simulink model "KinematicsComplianceIndependentSuspensionFront"  (R2026b)
settings: Solver=VariableStepAuto
undefined symbols (not defined in the file): PlntVehCGHgtAxl, PlntVehTrckWdth, PlntWhlNumFrnt
libraries: autolibsharedcommon x6, autolibutils x3, matrix_library x2, vehdynlibsuspension x1
(part 1 of 2)
settings Model: ModifiedByFormat=The MathWorks, Inc.  Creator=The MathWorks, Inc.  LastModifiedBy=The MathWorks, Inc.
settings OptimizationCC: ReuseModelBlockBuffer=off
settings DebuggingCC: SubsystemReferenceDiagnosticForUnitTest=warning
settings RTWCC: LargeConstantGeneration=WriteOnlyDNNConstantsToDataFiles

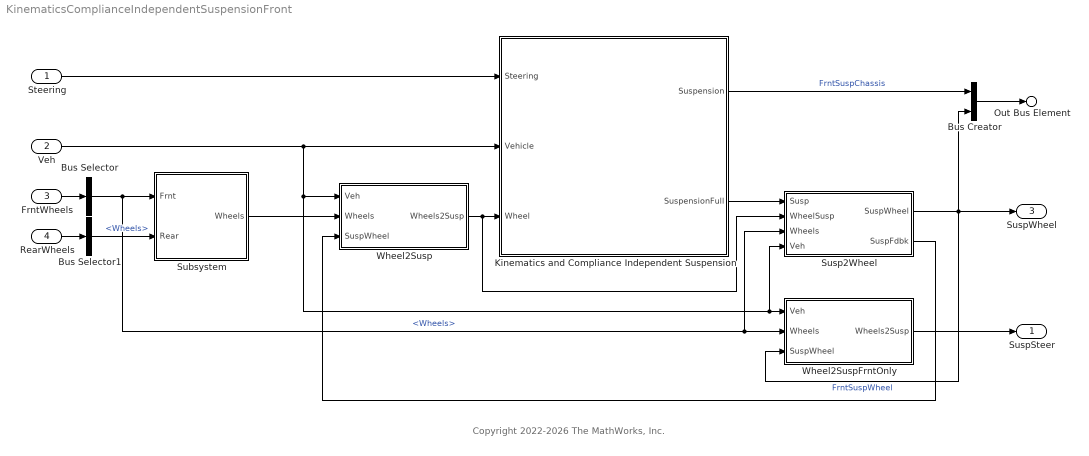
== system KinematicsComplianceIndependentSuspensionFront ==
  note: Copyright 2022-2026 The MathWorks, Inc.
  Steering : Inport
  Veh : Inport  Port=2
  FrntWheels : Inport  Port=3
  RearWheels : Inport  Port=4
  Bus Creator : BusCreator  Inputs=2
  Bus Selector : BusSelector  OutputSignals=Wheels
  Bus Selector1 : BusSelector  OutputSignals=Wheels
  Kinematics and Compliance Independent Suspension : Subsystem  VariantControl=Kinematics and Compliance Independent Suspension
      mask Display: image('suspkandc.png');
  Subsystem : Subsystem
  Susp2Wheel : Subsystem
  Wheel2Susp : Subsystem
  Wheel2SuspFrntOnly : Subsystem
  SuspSteer : Outport
  Out Bus Element : Outport  Port=2  PortName=FrntSusp
  SuspWheel : Outport  Port=3
  wires:
  Veh/1 -> Kinematics and Compliance Independent Suspension/2(Vehicle), Susp2Wheel/4(Veh), Wheel2SuspFrntOnly/1(Veh), Wheel2Susp/1(Veh)
  Susp2Wheel/1(SuspWheel) -> Wheel2SuspFrntOnly/3(SuspWheel), Bus Creator/2, SuspWheel/1  "FrntSuspWheel"
  Subsystem/1(Wheels) -> Wheel2Susp/2(Wheels)
  Kinematics and Compliance Independent Suspension/1(Suspension) -> Bus Creator/1  "FrntSuspChassis"
  Wheel2Susp/1(Wheels2Susp) -> Susp2Wheel/2(WheelSusp), Kinematics and Compliance Independent Suspension/3(Wheel)
  Steering/1 -> Kinematics and Compliance Independent Suspension/1(Steering)
  Bus Selector/1 -> Susp2Wheel/3(Wheels), Wheel2SuspFrntOnly/2(Wheels), Subsystem/1(Frnt)  "<Wheels>"
  RearWheels/1 -> Bus Selector1/1
  FrntWheels/1 -> Bus Selector/1
  Bus Selector1/1 -> Subsystem/2(Rear)  "<Wheels>"
  Bus Creator/1 -> Out Bus Element/1
  Susp2Wheel/2(SuspFdbk) -> Wheel2Susp/3(SuspWheel)
  Kinematics and Compliance Independent Suspension/2(SuspensionFull) -> Susp2Wheel/1(Susp)
  Wheel2SuspFrntOnly/1(Wheels2Susp) -> SuspSteer/1

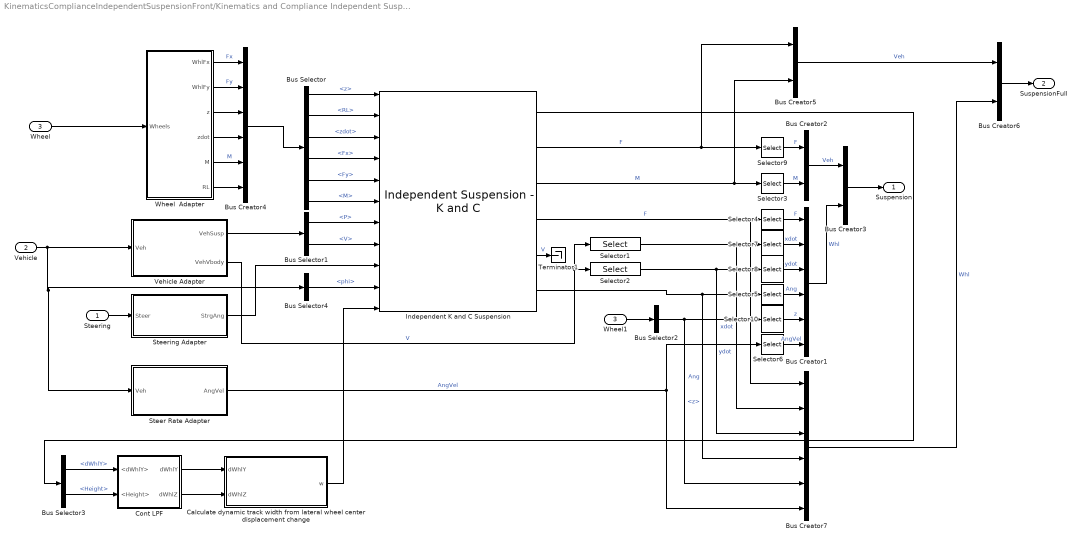
== system KinematicsComplianceIndependentSuspensionFront/Kinematics and Compliance Independent Suspension ==
  Steering : Inport
  Vehicle : Inport  Port=2
  Wheel : Inport  Port=3
  Bus Creator1 : BusCreator  Inputs=6
  Bus Creator{2..3,5..6} (4 alike) : BusCreator  Inputs=2
  Bus Creator4 : BusCreator  Inputs=6
  Bus Creator7 : BusCreator  Inputs=6
  Bus Selector : BusSelector  OutputSignals=z,RL,zdot,Fx,Fy,M
  Bus Selector1 : BusSelector  OutputSignals=P,V
  Bus Selector2 : BusSelector  OutputSignals=SuspFrame.z
  Bus Selector3 : BusSelector  OutputSignals=dWhlY,Height
  Bus Selector4 : BusSelector  OutputSignals=InertFrm.Cg.Ang.phi
  Calculate dynamic track width from lateral wheel center displacement change : Subsystem  mask{w=PlntVehTrckWdth}
      mask prompts: w "vdynblks:vehdynVehBody6Dof:blkPrm_w"
      mask DialogControl w Prompt: Track widths [front, rear], w [m]:
  Cont LPF : Subsystem
  Independent K and C Suspension : vehdynlibsuspension/Independent Suspension - K and C  ActiveDampEn=off  NumAxl=2  NumWhlsByAxl=[2 2]  StrgEnByAxl=[1 0]  AntiSwayEnByAxl=[1 1]  WhlNumVec="[1  2  1  2]"  AxleNumVec="[1  1  2  2]"  SuspTypesByAxle="[1  1]"  SuspImage=suspkandc.png  IdealSuspEn=on  IdealSuspAxles="[1  2]"  tanTheta_FL=[0 0 0]  tanTheta_FR=[0 0 0]  tanTheta_RL=[0 0 0]  tanTheta_RR=[0 0 0]  SteerSign=1  LongitudinalSign=1  LateralSign=1  VerticalSign=1  WhlMzSign=1  tanTheta_SVSA_WC_FL=1  tanTheta_SVSA_WC_FR=1  tanTheta_SVSA_WC_RL=1  tanTheta_SVSA_WC_RR=1  tanTheta_SVSA_CP_FL=1  tanTheta_SVSA_CP_FR=1  tanTheta_SVSA_CP_RL=1  tanTheta_SVSA_CP_RR=1  SuspType=Independent front and rear  DrivetrainType=FWD  StrPlusDirection=Right  XPlusDirection=Front  YPlusDirection=Right  ZPlusDirection=Up  WhlMzDirection=Counter-clockwise  ShockType=Constant  ShckFrcVsCompRate=PlntSpKCShckFrcVsCompRate  MotRatios=PlntSpKCMotRatios  BumpSteer=PlntSpKCBumpSteer  BumpCamber=PlntSpKCBumpCamber  BumpCaster=PlntSpKCBumpCaster  LatWhlCtrDisp=PlntSpKCLatWhlCtrDisp  LngWhlCtrDisp=PlntSpKCLngWhlCtrDisp  NrmlWhlRates=PlntSpKCNrmlWhlRates  NrmlWhlFrcOff=PlntSpKCNrmlWhlFrcOff  RollSteer=[0 0 0 0]  RollCamber=[0 0 0 0]  RollCaster=[0 0 0 0]  RollStiffArb=PlntSpKCRollStiffArb  RollStiffNoArb=PlntSpKCRollStiffNoArb  RollStiffArbFrnt=800  RollStiffNoArbFrnt=0  RollStiffNoTwstRear=0  CambVsSteerAng=PlntSpKCCambVsSteerAng  CastVsSteerAng=PlntSpKCCastVsSteerAng  LngSteerCompl=PlntSpKCLngSteerCompl  LngCambCompl=PlntSpKCLngCambCompl  LngCastCompl=PlntSpKCLngCastCompl  LngWhlCtrCompl=PlntSpKCLngWhlCtrCompl  LatWhlCtrComplLng=PlntSpKCLatWhlCtrComplLng  LatSteerCompl=PlntSpKCLatSteerCompl  LatCambCompl=PlntSpKCLatCambCompl  LatWhlCtrComplLat=PlntSpKCLatWhlCtrComplLat  LatSteerComplOpp=PlntSpKCLatSteerCompl  LatCambComplOpp=PlntSpKCLatCambCompl  LatWhlCtrComplLatOpp=PlntSpKCLatWhlCtrComplLat  AlgnTrqSteerCompl=PlntSpKCAlgnTrqSteerCompl  AlgnTrqCambCompl=PlntSpKCAlgnTrqCambCompl  VrtLdTrnsfr=PlntSpKCVrtLdTrnsfr  LatSteerComplPar=struct('FL',[-2. -1.;0 0;2. 1.],'FR',[-2. 1.;0 0;2. -1.],'RL',[-2. -1.;0 0;2. 1.],'RR',[-2. 1.;0 0;2. -1.])  LatCambComplPar=struct('FL',[-2. -1.;0 0;2. 1.],'FR',[-2. 1.;0 0;2. -1.],'RL',[-2. -1.;0 0;2. 1.],'RR',[-2. 1.;0 0;2. -1.])  LatWhlCtrComplLatPar=struct('FL',[-2. -5.;0 0;2. 5.],'FR',[-2. 5.;0 0;2. -5.],'RL',[-2. -5.;0 0;2. 5.],'RR',[-2. 5.;0 0;2. -5.])  StatToe=PlntSpKCStatToe  StatCamber=PlntSpKCStatCamber  StatCaster=PlntSpKCStatCaster  StatLdWhlR=PlntSpStatLdWhlR  MappedSuspEn=off  RollParamEn=off
  Selector1 : Selector  NumberOfDimensions=2  IndexOptions=Index vector (dialog),Select all  Indices=1,1  OutputSizes=1,1
  Selector10 : Selector  InputPortWidth=4  IndexOptions=Index vector (dialog)  Indices=[1 2]  OutputSizes=1
  Selector2 : Selector  NumberOfDimensions=2  IndexOptions=Index vector (dialog),Select all  Indices=2,1  OutputSizes=1,1
  Selector{3..6,9} (5 alike) : Selector  NumberOfDimensions=2  InputPortWidth=4  IndexOptions=Index vector (dialog),Index vector (dialog)  Indices=[1 2 3],[1 2]  OutputSizes=1,1
  Selector7 : Selector  InputPortWidth=4  IndexOptions=Index vector (dialog)  Indices=[1 2]  OutputSizes=1
  Selector8 : Selector  InputPortWidth=4  IndexOptions=Index vector (dialog)  Indices=[1 2]  OutputSizes=1
  Steer Rate Adapter : Subsystem
  Steering Adapter : Subsystem
  Terminator1 : Terminator
  Vehicle Adapter : Subsystem
  Wheel  Adapter : Subsystem
  Wheel1 : InportShadow  Port=3
  Suspension : Outport  VectorParamsAs1DForOutWhenUnconnected=off
  SuspensionFull : Outport  Port=2  VectorParamsAs1DForOutWhenUnconnected=off
  wires:
  Bus Creator6/1 -> SuspensionFull/1
  Bus Creator7/1 -> Bus Creator6/2  "Whl"
  Bus Creator5/1 -> Bus Creator6/1  "Veh"
  Selector6/1 -> Bus Creator1/6  "AngVel"
  Selector10/1 -> Bus Creator1/5  "z"
  Selector5/1 -> Bus Creator1/4  "Ang"
  Selector8/1 -> Bus Creator1/3  "ydot"
  Selector7/1 -> Bus Creator1/2  "xdot"
  Selector4/1 -> Bus Creator1/1  "F"
  Selector3/1 -> Bus Creator2/2  "M"
  Selector9/1 -> Bus Creator2/1  "F"
  Bus Creator3/1 -> Suspension/1
  Bus Creator1/1 -> Bus Creator3/2  "Whl"
  Bus Selector1/2 -> Independent K and C Suspension/8  "<V>"
  Bus Selector/6 -> Independent K and C Suspension/6  "<M>"
  Bus Selector/5 -> Independent K and C Suspension/5  "<Fy>"
  Steering/1 -> Steering Adapter/1(Steer)
  Bus Selector/3 -> Independent K and C Suspension/3  "<zdot>"
  Bus Selector/4 -> Independent K and C Suspension/4  "<Fx>"
  Vehicle/1 -> Vehicle Adapter/1(Veh), Bus Selector4/1, Steer Rate Adapter/1(Veh)
  Vehicle Adapter/1(VehSusp) -> Bus Selector1/1
  Independent K and C Suspension/3 -> Selector3/1, Bus Creator5/2  "M"
  Wheel  Adapter/2(WhlFy) -> Bus Creator4/2  "Fy"
  Wheel  Adapter/1(WhlFx) -> Bus Creator4/1  "Fx"
  Wheel/1 -> Wheel  Adapter/1(Wheels)
  Wheel  Adapter/3(z) -> Bus Creator4/3
  Wheel  Adapter/4(zdot) -> Bus Creator4/4
  Wheel  Adapter/5(M) -> Bus Creator4/5  "M"
  Wheel  Adapter/6(RL) -> Bus Creator4/6
  Bus Selector/2 -> Independent K and C Suspension/2  "<RL>"
  Selector1/1 -> Selector7/1, Bus Creator7/2  "xdot"
  Selector2/1 -> Selector8/1, Bus Creator7/3  "ydot"
  Bus Selector1/1 -> Independent K and C Suspension/7  "<P>"
  Bus Selector/1 -> Independent K and C Suspension/1  "<z>"
  Independent K and C Suspension/4 -> Selector4/1, Bus Creator7/1  "F"
  Independent K and C Suspension/6 -> Selector5/1, Bus Creator7/4  "Ang"
  Vehicle Adapter/2(VehVbody) -> Selector1/1, Selector2/1  "V"
  Independent K and C Suspension/2 -> Selector9/1, Bus Creator5/1  "F"
  Bus Creator2/1 -> Bus Creator3/1  "Veh"
  Bus Creator4/1 -> Bus Selector/1
  Steer Rate Adapter/1(AngVel) -> Selector6/1, Bus Creator7/6  "AngVel"
  Steering Adapter/1(StrgAng) -> Independent K and C Suspension/9
  Independent K and C Suspension/1 -> Bus Selector3/1
  Independent K and C Suspension/5 -> Terminator1/1  "V"
  Bus Selector2/1 -> Selector10/1, Bus Creator7/5  "<z>"
  Wheel1/1 -> Bus Selector2/1
  Bus Selector4/1 -> Independent K and C Suspension/10  "<phi>"
  Calculate dynamic track width from lateral wheel center displacement change/1(w) -> Independent K and C Suspension/11
  Bus Selector3/1 -> Cont LPF/1(<dWhlY>)  "<dWhlY>"
  Bus Selector3/2 -> Cont LPF/2(<Height>)  "<Height>"
  Cont LPF/1(dWhlY) -> Calculate dynamic track width from lateral wheel center displacement change/1(dWhlY)
  Cont LPF/2(dWhlZ) -> Calculate dynamic track width from lateral wheel center displacement change/2(dWhlZ)

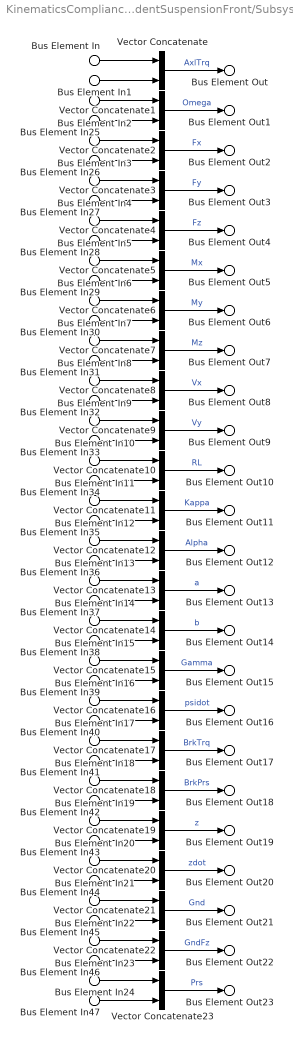
== system KinematicsComplianceIndependentSuspensionFront/Subsystem ==
  Bus Element In : Inport  PortName=Frnt  Element=AxlTrq
  Bus Element In2 : Inport  PortName=Frnt  Element=Omega
  Bus Element In3 : Inport  PortName=Frnt  Element=Fx
  Bus Element In4 : Inport  PortName=Frnt  Element=Fy
  Bus Element In5 : Inport  PortName=Frnt  Element=Fz
  Bus Element In6 : Inport  PortName=Frnt  Element=Mx
  Bus Element In7 : Inport  PortName=Frnt  Element=My
  Bus Element In8 : Inport  PortName=Frnt  Element=Mz
  Bus Element In9 : Inport  PortName=Frnt  Element=Vx
  Bus Element In10 : Inport  PortName=Frnt  Element=Vy
  Bus Element In11 : Inport  PortName=Frnt  Element=RL
  Bus Element In12 : Inport  PortName=Frnt  Element=Kappa
  Bus Element In13 : Inport  PortName=Frnt  Element=Alpha
  Bus Element In14 : Inport  PortName=Frnt  Element=a
  Bus Element In15 : Inport  PortName=Frnt  Element=b
  Bus Element In16 : Inport  PortName=Frnt  Element=Gamma
  Bus Element In17 : Inport  PortName=Frnt  Element=psidot
  Bus Element In18 : Inport  PortName=Frnt  Element=BrkTrq
  Bus Element In19 : Inport  PortName=Frnt  Element=BrkPrs
  Bus Element In20 : Inport  PortName=Frnt  Element=z
  Bus Element In21 : Inport  PortName=Frnt  Element=zdot
  Bus Element In22 : Inport  PortName=Frnt  Element=Gnd
  Bus Element In23 : Inport  PortName=Frnt  Element=GndFz
  Bus Element In24 : Inport  PortName=Frnt  Element=Prs
  Bus Element In1 : Inport  Port=2  PortName=Rear  Element=AxlTrq
  Bus Element In25 : Inport  Port=2  PortName=Rear  Element=Omega
  Bus Element In26 : Inport  Port=2  PortName=Rear  Element=Fx
  Bus Element In27 : Inport  Port=2  PortName=Rear  Element=Fy
  Bus Element In28 : Inport  Port=2  PortName=Rear  Element=Fz
  Bus Element In29 : Inport  Port=2  PortName=Rear  Element=Mx
  Bus Element In30 : Inport  Port=2  PortName=Rear  Element=My
  Bus Element In31 : Inport  Port=2  PortName=Rear  Element=Mz
  Bus Element In32 : Inport  Port=2  PortName=Rear  Element=Vx
  Bus Element In33 : Inport  Port=2  PortName=Rear  Element=Vy
  Bus Element In34 : Inport  Port=2  PortName=Rear  Element=RL
  Bus Element In35 : Inport  Port=2  PortName=Rear  Element=Kappa
  Bus Element In36 : Inport  Port=2  PortName=Rear  Element=Alpha
  Bus Element In37 : Inport  Port=2  PortName=Rear  Element=a
  Bus Element In38 : Inport  Port=2  PortName=Rear  Element=b
  Bus Element In39 : Inport  Port=2  PortName=Rear  Element=Gamma
  Bus Element In40 : Inport  Port=2  PortName=Rear  Element=psidot
  Bus Element In41 : Inport  Port=2  PortName=Rear  Element=BrkTrq
  Bus Element In42 : Inport  Port=2  PortName=Rear  Element=BrkPrs
  Bus Element In43 : Inport  Port=2  PortName=Rear  Element=z
  Bus Element In44 : Inport  Port=2  PortName=Rear  Element=zdot
  Bus Element In45 : Inport  Port=2  PortName=Rear  Element=Gnd
  Bus Element In46 : Inport  Port=2  PortName=Rear  Element=GndFz
  Bus Element In47 : Inport  Port=2  PortName=Rear  Element=Prs
  Vector Concatenate{,1..23} (24 alike) : Concatenate
  Bus Element Out : Outport  PortName=Wheels  Element=AxlTrq
  Bus Element Out1 : Outport  PortName=Wheels  Element=Omega
  Bus Element Out2 : Outport  PortName=Wheels  Element=Fx
  Bus Element Out3 : Outport  PortName=Wheels  Element=Fy
  Bus Element Out4 : Outport  PortName=Wheels  Element=Fz
  Bus Element Out5 : Outport  PortName=Wheels  Element=Mx
  Bus Element Out6 : Outport  PortName=Wheels  Element=My
  Bus Element Out7 : Outport  PortName=Wheels  Element=Mz
  Bus Element Out8 : Outport  PortName=Wheels  Element=Vx
  Bus Element Out9 : Outport  PortName=Wheels  Element=Vy
  Bus Element Out10 : Outport  PortName=Wheels  Element=RL
  Bus Element Out11 : Outport  PortName=Wheels  Element=Kappa
  Bus Element Out12 : Outport  PortName=Wheels  Element=Alpha
  Bus Element Out13 : Outport  PortName=Wheels  Element=a
  Bus Element Out14 : Outport  PortName=Wheels  Element=b
  Bus Element Out15 : Outport  PortName=Wheels  Element=Gamma
  Bus Element Out16 : Outport  PortName=Wheels  Element=psidot
  Bus Element Out17 : Outport  PortName=Wheels  Element=BrkTrq
  Bus Element Out18 : Outport  PortName=Wheels  Element=BrkPrs
  Bus Element Out19 : Outport  PortName=Wheels  Element=z
  Bus Element Out20 : Outport  PortName=Wheels  Element=zdot
  Bus Element Out21 : Outport  PortName=Wheels  Element=Gnd
  Bus Element Out22 : Outport  PortName=Wheels  Element=GndFz
  Bus Element Out23 : Outport  PortName=Wheels  Element=Prs
  wires:
  Vector Concatenate23/1 -> Bus Element Out23/1  "Prs"
  Vector Concatenate22/1 -> Bus Element Out22/1  "GndFz"
  Vector Concatenate21/1 -> Bus Element Out21/1  "Gnd"
  Vector Concatenate20/1 -> Bus Element Out20/1  "zdot"
  Vector Concatenate19/1 -> Bus Element Out19/1  "z"
  Vector Concatenate18/1 -> Bus Element Out18/1  "BrkPrs"
  Vector Concatenate17/1 -> Bus Element Out17/1  "BrkTrq"
  Vector Concatenate16/1 -> Bus Element Out16/1  "psidot"
  Vector Concatenate15/1 -> Bus Element Out15/1  "Gamma"
  Vector Concatenate14/1 -> Bus Element Out14/1  "b"
  Vector Concatenate13/1 -> Bus Element Out13/1  "a"
  Vector Concatenate12/1 -> Bus Element Out12/1  "Alpha"
  Vector Concatenate11/1 -> Bus Element Out11/1  "Kappa"
  Vector Concatenate10/1 -> Bus Element Out10/1  "RL"
  Vector Concatenate9/1 -> Bus Element Out9/1  "Vy"
  Vector Concatenate8/1 -> Bus Element Out8/1  "Vx"
  Vector Concatenate7/1 -> Bus Element Out7/1  "Mz"
  Vector Concatenate6/1 -> Bus Element Out6/1  "My"
  Vector Concatenate5/1 -> Bus Element Out5/1  "Mx"
  Vector Concatenate4/1 -> Bus Element Out4/1  "Fz"
  Vector Concatenate3/1 -> Bus Element Out3/1  "Fy"
  Vector Concatenate2/1 -> Bus Element Out2/1  "Fx"
  Vector Concatenate1/1 -> Bus Element Out1/1  "Omega"
  Vector Concatenate/1 -> Bus Element Out/1  "AxlTrq"
  Bus Element In47/1 -> Vector Concatenate23/2
  Bus Element In24/1 -> Vector Concatenate23/1
  Bus Element In46/1 -> Vector Concatenate22/2
  Bus Element In23/1 -> Vector Concatenate22/1
  Bus Element In45/1 -> Vector Concatenate21/2
  Bus Element In22/1 -> Vector Concatenate21/1
  Bus Element In44/1 -> Vector Concatenate20/2
  Bus Element In21/1 -> Vector Concatenate20/1
  Bus Element In43/1 -> Vector Concatenate19/2
  Bus Element In20/1 -> Vector Concatenate19/1
  Bus Element In42/1 -> Vector Concatenate18/2
  Bus Element In19/1 -> Vector Concatenate18/1
  Bus Element In41/1 -> Vector Concatenate17/2
  Bus Element In18/1 -> Vector Concatenate17/1
  Bus Element In40/1 -> Vector Concatenate16/2
  Bus Element In17/1 -> Vector Concatenate16/1
  Bus Element In39/1 -> Vector Concatenate15/2
  Bus Element In16/1 -> Vector Concatenate15/1
  Bus Element In38/1 -> Vector Concatenate14/2
  Bus Element In15/1 -> Vector Concatenate14/1
  Bus Element In37/1 -> Vector Concatenate13/2
  Bus Element In14/1 -> Vector Concatenate13/1
  Bus Element In36/1 -> Vector Concatenate12/2
  Bus Element In13/1 -> Vector Concatenate12/1
  Bus Element In35/1 -> Vector Concatenate11/2
  Bus Element In12/1 -> Vector Concatenate11/1
  Bus Element In34/1 -> Vector Concatenate10/2
  Bus Element In11/1 -> Vector Concatenate10/1
  Bus Element In33/1 -> Vector Concatenate9/2
  Bus Element In10/1 -> Vector Concatenate9/1
  Bus Element In32/1 -> Vector Concatenate8/2
  Bus Element In9/1 -> Vector Concatenate8/1
  Bus Element In31/1 -> Vector Concatenate7/2
  Bus Element In8/1 -> Vector Concatenate7/1
  Bus Element In30/1 -> Vector Concatenate6/2
  Bus Element In7/1 -> Vector Concatenate6/1
  Bus Element In29/1 -> Vector Concatenate5/2
  Bus Element In6/1 -> Vector Concatenate5/1
  Bus Element In28/1 -> Vector Concatenate4/2
  Bus Element In5/1 -> Vector Concatenate4/1
  Bus Element In27/1 -> Vector Concatenate3/2
  Bus Element In4/1 -> Vector Concatenate3/1
  Bus Element In26/1 -> Vector Concatenate2/2
  Bus Element In3/1 -> Vector Concatenate2/1
  Bus Element In25/1 -> Vector Concatenate1/2
  Bus Element In2/1 -> Vector Concatenate1/1
  Bus Element In1/1 -> Vector Concatenate/2
  Bus Element In/1 -> Vector Concatenate/1

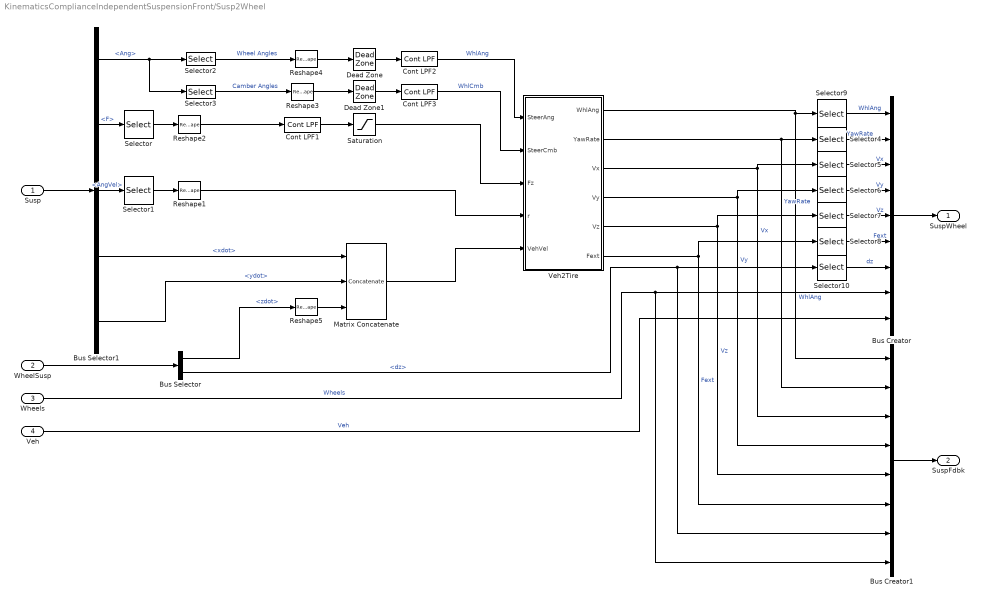
== system KinematicsComplianceIndependentSuspensionFront/Susp2Wheel ==
  Susp : Inport
  WheelSusp : Inport  Port=2
  Wheels : Inport  Port=3
  Veh : Inport  Port=4
  Bus Creator : BusCreator  Inputs=9
  Bus Creator1 : BusCreator  Inputs=8
  Bus Selector : BusSelector  OutputSignals=SuspFrame.zdot,SuspFrame.dz
  Bus Selector1 : BusSelector  OutputSignals=Whl.Ang,Whl.F,Whl.AngVel,Whl.xdot,Whl.ydot
  Cont LPF1 : autolibutils/Cont LPF  wc=100*2*pi  AbsoluteTolerance=auto  aMode=2
  Cont LPF2 : autolibutils/Cont LPF  wc=100*2*pi  AbsoluteTolerance=auto  aMode=2
  Cont LPF3 : autolibutils/Cont LPF  wc=100*2*pi  AbsoluteTolerance=auto  aMode=2
  Dead Zone : DeadZone  LowerValue=-pi/360/2  UpperValue=pi/360/2  ZeroCross=off
  Dead Zone1 : DeadZone  LowerValue=-pi/360/2  UpperValue=pi/360/2  ZeroCross=off
  Matrix Concatenate : Concatenate  NumInputs=3  Mode=Multidimensional array
  Reshape{1..4} (4 alike) : Reshape
  Reshape5 : Reshape  OutputDimensionality=Row vector (2-D)
  Saturation : Saturate  UpperLimit=inf  LowerLimit=-10*9.81*2000  ZeroCross=off
  Selector : Selector  NumberOfDimensions=2  InputPortWidth=3  IndexOptions=Index vector (dialog),Select all  Indices=[3],1  OutputSizes=1,1
  Selector1 : Selector  NumberOfDimensions=2  InputPortWidth=1  IndexOptions=Index vector (dialog),Select all  Indices=[3],1  OutputSizes=1,1
  Selector{4..8,10} (6 alike) : Selector  InputPortWidth=4  IndexOptions=Index vector (dialog)  Indices=[1 2]  OutputSizes=1
  Selector2 : Selector  NumberOfDimensions=2  InputPortWidth=3  IndexOptions=Index vector (dialog),Select all  Indices=3,1  OutputSizes=1,1
  Selector3 : Selector  NumberOfDimensions=2  InputPortWidth=3  IndexOptions=Index vector (dialog),Select all  Indices=1,1  OutputSizes=1,1
  Selector9 : Selector  NumberOfDimensions=2  InputPortWidth=4  IndexOptions=Index vector (dialog),Index vector (dialog)  Indices=[1 2 3],[1 2]  OutputSizes=1,1
  Veh2Tire : Subsystem
  SuspWheel : Outport
  SuspFdbk : Outport  Port=2
  wires:
  Bus Creator1/1 -> SuspFdbk/1
  Selector10/1 -> Bus Creator/7  "dz"
  Selector9/1 -> Bus Creator/1  "WhlAng"
  Selector8/1 -> Bus Creator/6  "Fext"
  Selector7/1 -> Bus Creator/5  "Vz"
  Selector6/1 -> Bus Creator/4  "Vy"
  Selector5/1 -> Bus Creator/3  "Vx"
  Selector4/1 -> Bus Creator/2  "YawRate"
  Wheels/1 -> Bus Creator1/8, Bus Creator/8  "Wheels"
  Bus Creator/1 -> SuspWheel/1
  Bus Selector/1 -> Reshape5/1  "<zdot>"
  Veh2Tire/3(Vx) -> Selector5/1, Bus Creator1/3  "Vx"
  Veh2Tire/4(Vy) -> Selector6/1, Bus Creator1/4  "Vy"
  Susp/1 -> Bus Selector1/1
  Veh2Tire/5(Vz) -> Selector7/1, Bus Creator1/5  "Vz"
  Reshape5/1 -> Matrix Concatenate/3
  WheelSusp/1 -> Bus Selector/1
  Selector/1 -> Reshape2/1
  Matrix Concatenate/1 -> Veh2Tire/5(VehVel)
  Selector1/1 -> Reshape1/1
  Veh2Tire/6(Fext) -> Selector8/1, Bus Creator1/6  "Fext"
  Bus Selector1/5 -> Matrix Concatenate/2  "<ydot>"
  Bus Selector1/3 -> Selector1/1  "<AngVel>"
  Bus Selector1/4 -> Matrix Concatenate/1  "<xdot>"
  Veh2Tire/1(WhlAng) -> Selector9/1, Bus Creator1/1  "WhlAng"
  Reshape2/1 -> Cont LPF1/1
  Reshape1/1 -> Veh2Tire/4(r)
  Bus Selector1/2 -> Selector/1  "<F>"
  Veh2Tire/2(YawRate) -> Selector4/1, Bus Creator1/2  "YawRate"
  Bus Selector/2 -> Bus Creator1/7, Selector10/1  "<dz>"
  Veh/1 -> Bus Creator/9  "Veh"
  Cont LPF1/1 -> Saturation/1
  Selector3/1 -> Reshape3/1  "Camber Angles"
  Selector2/1 -> Reshape4/1  "Wheel Angles"
  Reshape4/1 -> Dead Zone/1
  Dead Zone1/1 -> Cont LPF3/1
  Dead Zone/1 -> Cont LPF2/1
  Cont LPF2/1 -> Veh2Tire/1(SteerAng)  "WhlAng"
  Saturation/1 -> Veh2Tire/3(Fz)
  Cont LPF3/1 -> Veh2Tire/2(SteerCmb)  "WhlCmb"
  Reshape3/1 -> Dead Zone1/1
  Bus Selector1/1 -> Selector3/1, Selector2/1  "<Ang>"

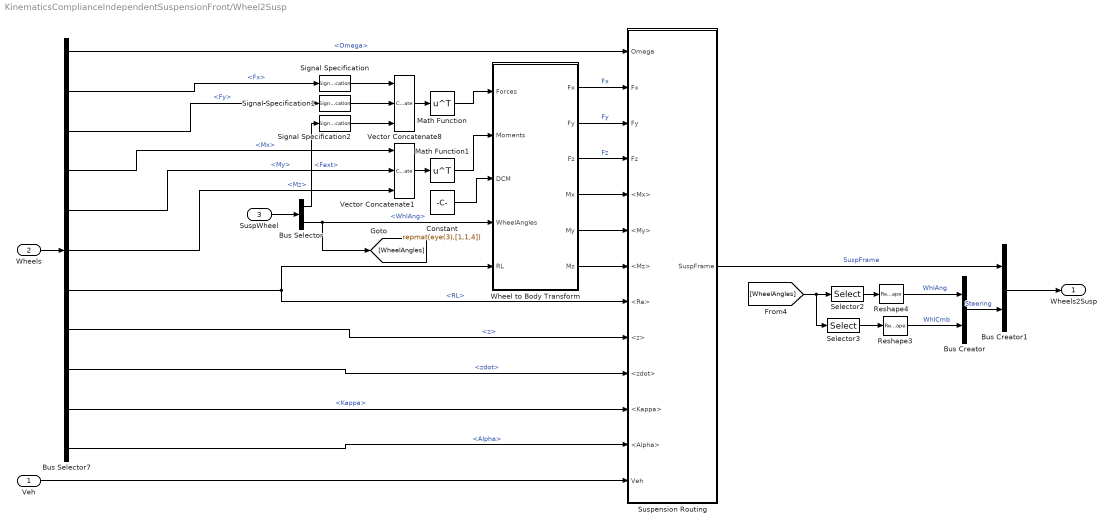
== system KinematicsComplianceIndependentSuspensionFront/Wheel2Susp ==
  Veh : Inport
  Wheels : Inport  Port=2
  SuspWheel : Inport  Port=3
  Bus Creator : BusCreator  Inputs=2
  Bus Creator1 : BusCreator  Inputs=2
  Bus Selector : BusSelector  OutputSignals=Fext,WhlAng
  Bus Selector7 : BusSelector  OutputSignals=Omega,Fx,Fy,Mx,My,Mz,RL,z,zdot,Kappa,Alpha
  Constant : Constant  Value=repmat(eye(3),[1,1,4])
  Math Function : Math  Operator=transpose  SignedPower=on
  Math Function1 : Math  Operator=transpose  SignedPower=on
  Reshape3 : Reshape
  Reshape4 : Reshape
  Selector2 : Selector  NumberOfDimensions=2  InputPortWidth=3  IndexOptions=Index vector (dialog),Select all  Indices=3,1  OutputSizes=1,1
  Selector3 : Selector  NumberOfDimensions=2  InputPortWidth=3  IndexOptions=Index vector (dialog),Select all  Indices=1,1  OutputSizes=1,1
  Signal Specification : SignalSpecification  Dimensions=4
  Signal Specification1 : SignalSpecification  Dimensions=4
  Signal Specification2 : SignalSpecification  Dimensions=4
  Suspension Routing : Subsystem
  Vector Concatenate1 : Concatenate  NumInputs=3  Mode=Multidimensional array  ConcatenateDimension=2
  Vector Concatenate8 : Concatenate  NumInputs=3  Mode=Multidimensional array  ConcatenateDimension=2
  Wheel to Body Transform : Subsystem
  Wheels2Susp : Outport  VectorParamsAs1DForOutWhenUnconnected=off
  wires:
  Bus Selector7/11 -> Suspension Routing/12(<Alpha>)  "<Alpha>"
  Bus Selector7/10 -> Suspension Routing/11(<Kappa>)  "<Kappa>"
  Bus Selector7/9 -> Suspension Routing/10(<zdot>)  "<zdot>"
  Bus Selector7/8 -> Suspension Routing/9(<z>)  "<z>"
  Bus Selector7/7 -> Suspension Routing/8(<Re>), Wheel to Body Transform/5(RL)  "<RL>"
  Bus Selector7/6 -> Vector Concatenate1/3  "<Mz>"
  Bus Selector7/5 -> Vector Concatenate1/2  "<My>"
  Bus Selector7/4 -> Vector Concatenate1/1  "<Mx>"
  Bus Selector7/3 -> Signal Specification1/1  "<Fy>"
  Bus Selector7/2 -> Signal Specification/1  "<Fx>"
  Bus Selector7/1 -> Suspension Routing/1(Omega)  "<Omega>"
  Constant/1 -> Wheel to Body Transform/3(DCM)
  Math Function1/1 -> Wheel to Body Transform/2(Moments)
  Vector Concatenate1/1 -> Math Function1/1
  Wheel to Body Transform/6(Mz) -> Suspension Routing/7(<Mz>)
  Wheel to Body Transform/5(My) -> Suspension Routing/6(<My>)
  Wheel to Body Transform/4(Mx) -> Suspension Routing/5(<Mx>)
  Selector3/1 -> Reshape3/1
  [WheelAngles] -> Selector3/1, Selector2/1
  Selector2/1 -> Reshape4/1
  Signal Specification2/1 -> Vector Concatenate8/3
  Bus Selector/1 -> Signal Specification2/1  "<Fext>"
  SuspWheel/1 -> Bus Selector/1
  Wheel to Body Transform/2(Fy) -> Suspension Routing/3(Fy)  "Fy"
  Wheel to Body Transform/1(Fx) -> Suspension Routing/2(Fx)  "Fx"
  Vector Concatenate8/1 -> Math Function/1
  Math Function/1 -> Wheel to Body Transform/1(Forces)
  Wheels/1 -> Bus Selector7/1
  Bus Selector/2 -> Wheel to Body Transform/4(WheelAngles), [WheelAngles]  "<WhlAng>"
  Wheel to Body Transform/3(Fz) -> Suspension Routing/4(Fz)  "Fz"
  Reshape4/1 -> Bus Creator/1  "WhlAng"
  Bus Creator1/1 -> Wheels2Susp/1
  Suspension Routing/1(SuspFrame) -> Bus Creator1/1  "SuspFrame"
  Reshape3/1 -> Bus Creator/2  "WhlCmb"
  Bus Creator/1 -> Bus Creator1/2  "Steering"
  Veh/1 -> Suspension Routing/13(Veh)
  Signal Specification/1 -> Vector Concatenate8/1
  Signal Specification1/1 -> Vector Concatenate8/2

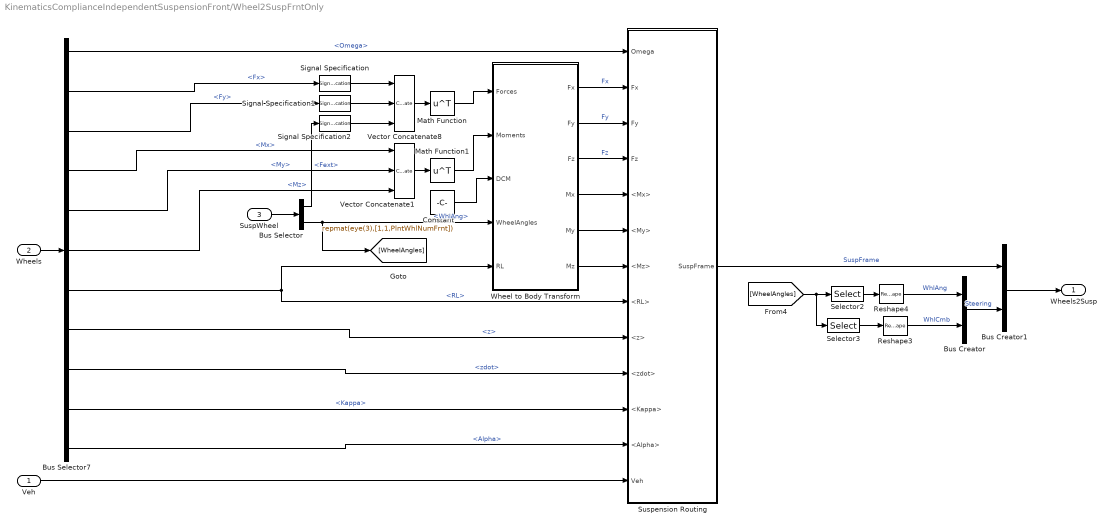
== system KinematicsComplianceIndependentSuspensionFront/Wheel2SuspFrntOnly ==
  Veh : Inport
  Wheels : Inport  Port=2
  SuspWheel : Inport  Port=3
  Bus Creator : BusCreator  Inputs=2
  Bus Creator1 : BusCreator  Inputs=2
  Bus Selector : BusSelector  OutputSignals=Fext,WhlAng
  Bus Selector7 : BusSelector  OutputSignals=Omega,Fx,Fy,Mx,My,Mz,RL,z,zdot,Kappa,Alpha
  Constant : Constant  Value=repmat(eye(3),[1,1,PlntWhlNumFrnt])
  Math Function : Math  Operator=transpose  SignedPower=on
  Math Function1 : Math  Operator=transpose  SignedPower=on
  Reshape3 : Reshape
  Reshape4 : Reshape
  Selector2 : Selector  NumberOfDimensions=2  InputPortWidth=3  IndexOptions=Index vector (dialog),Select all  Indices=3,1  OutputSizes=1,1
  Selector3 : Selector  NumberOfDimensions=2  InputPortWidth=3  IndexOptions=Index vector (dialog),Select all  Indices=1,1  OutputSizes=1,1
  Signal Specification : SignalSpecification  Dimensions=PlntWhlNumFrnt
  Signal Specification1 : SignalSpecification  Dimensions=PlntWhlNumFrnt
  Signal Specification2 : SignalSpecification  Dimensions=PlntWhlNumFrnt
  Suspension Routing : Subsystem
  Vector Concatenate1 : Concatenate  NumInputs=3  Mode=Multidimensional array  ConcatenateDimension=2
  Vector Concatenate8 : Concatenate  NumInputs=3  Mode=Multidimensional array  ConcatenateDimension=2
  Wheel to Body Transform : Subsystem
  Wheels2Susp : Outport  VectorParamsAs1DForOutWhenUnconnected=off
  wires:
  Bus Selector7/11 -> Suspension Routing/12(<Alpha>)  "<Alpha>"
  Bus Selector7/10 -> Suspension Routing/11(<Kappa>)  "<Kappa>"
  Bus Selector7/9 -> Suspension Routing/10(<zdot>)  "<zdot>"
  Bus Selector7/8 -> Suspension Routing/9(<z>)  "<z>"
  Bus Selector7/7 -> Suspension Routing/8(<RL>), Wheel to Body Transform/5(RL)  "<RL>"
  Bus Selector7/6 -> Vector Concatenate1/3  "<Mz>"
  Bus Selector7/5 -> Vector Concatenate1/2  "<My>"
  Bus Selector7/4 -> Vector Concatenate1/1  "<Mx>"
  Bus Selector7/3 -> Signal Specification1/1  "<Fy>"
  Bus Selector7/2 -> Signal Specification/1  "<Fx>"
  Bus Selector7/1 -> Suspension Routing/1(Omega)  "<Omega>"
  Constant/1 -> Wheel to Body Transform/3(DCM)
  Math Function1/1 -> Wheel to Body Transform/2(Moments)
  Vector Concatenate1/1 -> Math Function1/1
  Wheel to Body Transform/6(Mz) -> Suspension Routing/7(<Mz>)
  Wheel to Body Transform/5(My) -> Suspension Routing/6(<My>)
  Wheel to Body Transform/4(Mx) -> Suspension Routing/5(<Mx>)
  Selector3/1 -> Reshape3/1
  [WheelAngles] -> Selector3/1, Selector2/1
  Selector2/1 -> Reshape4/1
  Signal Specification2/1 -> Vector Concatenate8/3
  Bus Selector/1 -> Signal Specification2/1  "<Fext>"
  SuspWheel/1 -> Bus Selector/1
  Wheel to Body Transform/2(Fy) -> Suspension Routing/3(Fy)  "Fy"
  Wheel to Body Transform/1(Fx) -> Suspension Routing/2(Fx)  "Fx"
  Vector Concatenate8/1 -> Math Function/1
  Math Function/1 -> Wheel to Body Transform/1(Forces)
  Wheels/1 -> Bus Selector7/1
  Bus Selector/2 -> Wheel to Body Transform/4(WheelAngles), [WheelAngles]  "<WhlAng>"
  Wheel to Body Transform/3(Fz) -> Suspension Routing/4(Fz)  "Fz"
  Reshape4/1 -> Bus Creator/1  "WhlAng"
  Bus Creator1/1 -> Wheels2Susp/1
  Suspension Routing/1(SuspFrame) -> Bus Creator1/1  "SuspFrame"
  Reshape3/1 -> Bus Creator/2  "WhlCmb"
  Bus Creator/1 -> Bus Creator1/2  "Steering"
  Veh/1 -> Suspension Routing/13(Veh)
  Signal Specification/1 -> Vector Concatenate8/1
  Signal Specification1/1 -> Vector Concatenate8/2

== system KinematicsComplianceIndependentSuspensionFront/Kinematics and Compliance Independent Suspension/Calculate dynamic track width from lateral wheel center displacement change ==
  dWhlY : Inport
  dWhlZ : Inport  Port=2
  Front Track Calculation : Subsystem
  Gain : Gain  Gain=-1
  Rear Track Calculation : Subsystem
  Sign : Signum  ZeroCross=off
  Vector Concatenate : Concatenate
  w : Outport
  wires:
  dWhlZ/1 -> Gain/1
  dWhlY/1 -> Rear Track Calculation/1(dWhlY), Front Track Calculation/1(dWhlY)
  Vector Concatenate/1 -> w/1
  Front Track Calculation/1(w_front) -> Vector Concatenate/1
  Rear Track Calculation/1(w_rear) -> Vector Concatenate/2
  Sign/1 -> Rear Track Calculation/2(sign), Front Track Calculation/2(sign)
  Gain/1 -> Sign/1

== system KinematicsComplianceIndependentSuspensionFront/Kinematics and Compliance Independent Suspension/Cont LPF ==
  <dWhlY> : Inport
  <Height> : Inport  Port=2
  Demux : Demux
  Demux1 : Demux
  Transfer Fcn{,1..7} (8 alike) : TransferFcn  Denominator=[1/(100*2*pi) 1]
  Vector Concatenate : Concatenate  NumInputs=4
  Vector Concatenate1 : Concatenate  NumInputs=4
  dWhlY : Outport
  dWhlZ : Outport  Port=2
  wires:
  Transfer Fcn4/1 -> Vector Concatenate1/1
  Transfer Fcn7/1 -> Vector Concatenate1/4
  Transfer Fcn6/1 -> Vector Concatenate1/3
  Transfer Fcn5/1 -> Vector Concatenate1/2
  Transfer Fcn3/1 -> Vector Concatenate/4
  Transfer Fcn2/1 -> Vector Concatenate/3
  Transfer Fcn1/1 -> Vector Concatenate/2
  Transfer Fcn/1 -> Vector Concatenate/1
  <dWhlY>/1 -> Demux/1
  Vector Concatenate1/1 -> dWhlZ/1
  <Height>/1 -> Demux1/1
  Vector Concatenate/1 -> dWhlY/1
  Demux1/4 -> Transfer Fcn7/1
  Demux/3 -> Transfer Fcn2/1
  Demux/4 -> Transfer Fcn3/1
  Demux1/3 -> Transfer Fcn6/1
  Demux1/1 -> Transfer Fcn4/1
  Demux/2 -> Transfer Fcn1/1
  Demux/1 -> Transfer Fcn/1
  Demux1/2 -> Transfer Fcn5/1

== system KinematicsComplianceIndependentSuspensionFront/Kinematics and Compliance Independent Suspension/Steer Rate Adapter ==
  Veh : Inport
  Add : Sum
  Bus Selector3 : BusSelector  OutputSignals=BdyFrm.Cg.AngVel.r
  Constant : Constant  Value=zeros(1,4)  SampleTime=-1
  Matrix Concatenate : Concatenate  NumInputs=3  Mode=Multidimensional array
  Matrix Concatenate1 : Concatenate  NumInputs=3  Mode=Multidimensional array
  Reshape2 : Reshape  OutputDimensionality=Row vector (2-D)
  Reshape3 : Reshape  OutputDimensionality=Row vector (2-D)
  Reshape4 : Reshape  OutputDimensionality=Row vector (2-D)
  Selector3 : Selector  InputPortWidth=1  IndexOptions=Index vector (dialog)  Indices=[1 1 1 1]  OutputSizes=1
  SteerRates : Constant  Value=zeros(1,4)  SampleTime=-1
  AngVel : Outport  VectorParamsAs1DForOutWhenUnconnected=off
  wires:
  Reshape2/1 -> Matrix Concatenate1/1, Matrix Concatenate1/3, Matrix Concatenate1/2
  Constant/1 -> Reshape3/1
  Selector3/1 -> Reshape4/1
  Bus Selector3/1 -> Selector3/1  "<r>"
  Matrix Concatenate/1 -> Add/2
  SteerRates/1 -> Reshape2/1
  Reshape4/1 -> Matrix Concatenate/3
  Reshape3/1 -> Matrix Concatenate/2, Matrix Concatenate/1
  Matrix Concatenate1/1 -> Add/1
  Veh/1 -> Bus Selector3/1
  Add/1 -> AngVel/1  "AngVel"

== system KinematicsComplianceIndependentSuspensionFront/Kinematics and Compliance Independent Suspension/Steering Adapter ==
  Steer : Inport
  Reshape1 : Reshape  OutputDimensionality=Row vector (2-D)
  Selector : Selector  IndexOptions=Index vector (dialog)  Indices=[1 2]  OutputSizes=1
  StrgAng : Outport  VectorParamsAs1DForOutWhenUnconnected=off
  wires:
  Reshape1/1 -> StrgAng/1
  Steer/1 -> Selector/1
  Selector/1 -> Reshape1/1

== system KinematicsComplianceIndependentSuspensionFront/Kinematics and Compliance Independent Suspension/Vehicle Adapter ==
  Veh : Inport
  Bus Creator3 : BusCreator  Inputs=2
  Bus Selector1 : BusSelector  OutputSignals=InertFrm.FrntAxl.Lft.Disp.X,InertFrm.FrntAxl.Lft.Disp.Y,InertFrm.FrntAxl.Lft.Disp.Z,InertFrm.FrntAxl.Rght.Disp.X,InertFrm.FrntAxl.Rght.Disp.Y,InertFrm.FrntAxl.Rght.Disp.Z,InertFrm.RearAxl.Lft.Disp.X,InertFrm.RearAxl.Lft.Disp.Y,InertFrm.RearAxl.Lft.Disp.Z,InertFrm.RearAxl.Rght.Disp.X,InertFrm.RearAxl.Rght.Disp.Y,InertFrm.RearAxl.Rght.Disp.Z
  Bus Selector2 : BusSelector  OutputSignals=BdyFrm.FrntAxl.Lft.Vel.xdot,BdyFrm.FrntAxl.Lft.Vel.ydot,BdyFrm.FrntAxl.Lft.Vel.zdot,BdyFrm.FrntAxl.Rght.Vel.xdot,BdyFrm.FrntAxl.Rght.Vel.ydot,BdyFrm.FrntAxl.Rght.Vel.zdot,BdyFrm.RearAxl.Lft.Vel.xdot,BdyFrm.RearAxl.Lft.Vel.ydot,BdyFrm.RearAxl.Lft.Vel.zdot,BdyFrm.RearAxl.Rght.Vel.xdot,BdyFrm.RearAxl.Rght.Vel.ydot,BdyFrm.RearAxl.Rght.Vel.zdot
  Bus Selector3 : BusSelector  OutputSignals=InertFrm.FrntAxl.Lft.Vel.Xdot,InertFrm.FrntAxl.Lft.Vel.Ydot,InertFrm.FrntAxl.Lft.Vel.Zdot,InertFrm.FrntAxl.Rght.Vel.Xdot,InertFrm.FrntAxl.Rght.Vel.Ydot,InertFrm.FrntAxl.Rght.Vel.Zdot,InertFrm.RearAxl.Lft.Vel.Xdot,InertFrm.RearAxl.Lft.Vel.Ydot,InertFrm.RearAxl.Lft.Vel.Zdot,InertFrm.RearAxl.Rght.Vel.Xdot,InertFrm.RearAxl.Rght.Vel.Ydot,InertFrm.RearAxl.Rght.Vel.Zdot
  Inertial Frame CG to Axle Offset : Constant  Value=[zeros(2,4);PlntVehCGHgtAxl*ones(1,4)]  SampleTime=-1
  Mux1 : Mux  Inputs=12
  Mux2 : Mux  Inputs=12
  Mux3 : Mux  Inputs=12
  Reshape : Reshape  OutputDimensionality=Customize  OutputDimensions=[3,4]
  Reshape1 : Reshape  OutputDimensionality=Customize  OutputDimensions=[3,4]
  Reshape2 : Reshape  OutputDimensionality=Customize  OutputDimensions=[3,4]
  Sum : Sum  Inputs=|+-
  VehSusp : Outport  VectorParamsAs1DForOutWhenUnconnected=off
  VehVbody : Outport  Port=2  VectorParamsAs1DForOutWhenUnconnected=off
  wires:
  Veh/1 -> Bus Selector3/1, Bus Selector2/1, Bus Selector1/1
  Reshape2/1 -> VehVbody/1  "V"
  Bus Creator3/1 -> VehSusp/1  "Veh"
  Reshape/1 -> Sum/1
  Bus Selector1/1 -> Mux2/1  "<X>"
  Bus Selector1/2 -> Mux2/2  "<Y>"
  Bus Selector1/3 -> Mux2/3  "<Z>"
  Bus Selector1/4 -> Mux2/4  "<X>"
  Bus Selector1/5 -> Mux2/5  "<Y>"
  Bus Selector1/6 -> Mux2/6  "<Z>"
  Bus Selector1/7 -> Mux2/7  "<X>"
  Bus Selector1/8 -> Mux2/8  "<Y>"
  Bus Selector1/9 -> Mux2/9  "<Z>"
  Bus Selector1/10 -> Mux2/10  "<X>"
  Bus Selector1/11 -> Mux2/11  "<Y>"
  Bus Selector1/12 -> Mux2/12  "<Z>"
  Bus Selector2/1 -> Mux1/1  "<xdot>"
  Bus Selector2/2 -> Mux1/2  "<ydot>"
  Bus Selector2/3 -> Mux1/3  "<zdot>"
  Bus Selector2/4 -> Mux1/4  "<xdot>"
  Bus Selector2/5 -> Mux1/5  "<ydot>"
  Bus Selector2/6 -> Mux1/6  "<zdot>"
  Bus Selector2/7 -> Mux1/7  "<xdot>"
  Bus Selector2/8 -> Mux1/8  "<ydot>"
  Bus Selector2/9 -> Mux1/9  "<zdot>"
  Bus Selector2/10 -> Mux1/10  "<xdot>"
  Bus Selector2/11 -> Mux1/11  "<ydot>"
  Bus Selector2/12 -> Mux1/12  "<zdot>"
  Mux1/1 -> Reshape2/1
  Mux2/1 -> Reshape/1
  Inertial Frame CG to Axle Offset/1 -> Sum/2
  Sum/1 -> Bus Creator3/1  "P"
  Mux3/1 -> Reshape1/1
  Bus Selector3/12 -> Mux3/12  "<Zdot>"
  Bus Selector3/11 -> Mux3/11  "<Ydot>"
  Bus Selector3/10 -> Mux3/10  "<Xdot>"
  Bus Selector3/9 -> Mux3/9  "<Zdot>"
  Bus Selector3/8 -> Mux3/8  "<Ydot>"
  Bus Selector3/7 -> Mux3/7  "<Xdot>"
  Bus Selector3/6 -> Mux3/6  "<Zdot>"
  Bus Selector3/5 -> Mux3/5  "<Ydot>"
  Bus Selector3/4 -> Mux3/4  "<Xdot>"
  Bus Selector3/3 -> Mux3/3  "<Zdot>"
  Bus Selector3/2 -> Mux3/2  "<Ydot>"
  Bus Selector3/1 -> Mux3/1  "<Xdot>"
  Reshape1/1 -> Bus Creator3/2  "V"

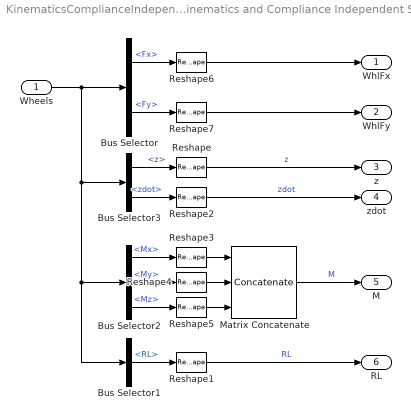
== system KinematicsComplianceIndependentSuspensionFront/Kinematics and Compliance Independent Suspension/Wheel  Adapter ==
  Wheels : Inport
  Bus Selector : BusSelector  OutputSignals=SuspFrame.Fx,SuspFrame.Fy
  Bus Selector1 : BusSelector  OutputSignals=SuspFrame.RL
  Bus Selector2 : BusSelector  OutputSignals=SuspFrame.Mx,SuspFrame.My,SuspFrame.Mz
  Bus Selector3 : BusSelector  OutputSignals=SuspFrame.z,SuspFrame.zdot
  Matrix Concatenate : Concatenate  NumInputs=3  Mode=Multidimensional array
  Reshape{,1..7} (8 alike) : Reshape  OutputDimensionality=Row vector (2-D)
  WhlFx : Outport  VectorParamsAs1DForOutWhenUnconnected=off
  WhlFy : Outport  Port=2  VectorParamsAs1DForOutWhenUnconnected=off
  z : Outport  Port=3  VectorParamsAs1DForOutWhenUnconnected=off
  zdot : Outport  Port=4  VectorParamsAs1DForOutWhenUnconnected=off
  M : Outport  Port=5  VectorParamsAs1DForOutWhenUnconnected=off
  RL : Outport  Port=6  VectorParamsAs1DForOutWhenUnconnected=off
  wires:
  Reshape7/1 -> WhlFy/1
  Reshape6/1 -> WhlFx/1
  Bus Selector/1 -> Reshape6/1  "<Fx>"
  Bus Selector/2 -> Reshape7/1  "<Fy>"
  Bus Selector3/1 -> Reshape/1  "<z>"
  Wheels/1 -> Bus Selector1/1, Bus Selector2/1, Bus Selector3/1, Bus Selector/1
  Bus Selector3/2 -> Reshape2/1  "<zdot>"
  Reshape2/1 -> zdot/1  "zdot"
  Bus Selector1/1 -> Reshape1/1  "<RL>"
  Reshape1/1 -> RL/1  "RL"
  Bus Selector2/1 -> Reshape3/1  "<Mx>"
  Bus Selector2/2 -> Reshape4/1  "<My>"
  Bus Selector2/3 -> Reshape5/1  "<Mz>"
  Reshape3/1 -> Matrix Concatenate/1
  Reshape4/1 -> Matrix Concatenate/2
  Reshape5/1 -> Matrix Concatenate/3
  Matrix Concatenate/1 -> M/1  "M"
  Reshape/1 -> z/1  "z"

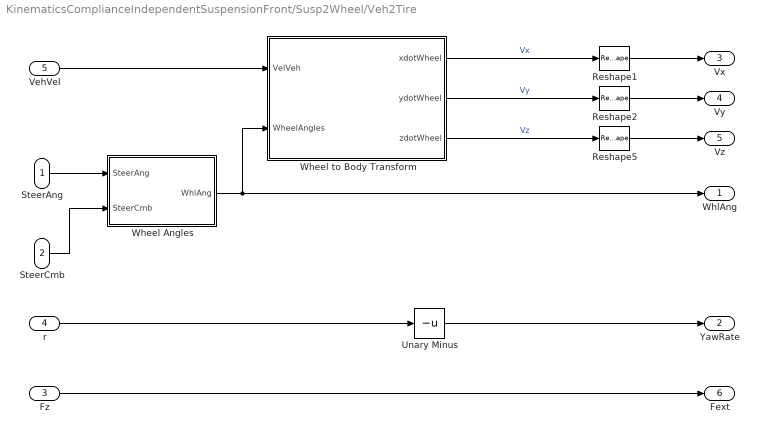
== system KinematicsComplianceIndependentSuspensionFront/Susp2Wheel/Veh2Tire ==
  SteerAng : Inport
  SteerCmb : Inport  Port=2
  Fz : Inport  Port=3
  r : Inport  Port=4
  VehVel : Inport  Port=5
  Reshape1 : Reshape
  Reshape2 : Reshape
  Reshape5 : Reshape
  Unary Minus : UnaryMinus
  Wheel Angles : Subsystem
  Wheel to Body Transform : Subsystem
  WhlAng : Outport  Unit=rad  VectorParamsAs1DForOutWhenUnconnected=off
  YawRate : Outport  Port=2  Unit=rad/s  VectorParamsAs1DForOutWhenUnconnected=off
  Vx : Outport  Port=3  Unit=m/s  VectorParamsAs1DForOutWhenUnconnected=off
  Vy : Outport  Port=4  Unit=m/s  VectorParamsAs1DForOutWhenUnconnected=off
  Vz : Outport  Port=5  Unit=m/s  VectorParamsAs1DForOutWhenUnconnected=off
  Fext : Outport  Port=6  Unit=N  VectorParamsAs1DForOutWhenUnconnected=off
  wires:
  Fz/1 -> Fext/1
  Wheel to Body Transform/1(xdotWheel) -> Reshape1/1  "Vx"
  Wheel to Body Transform/2(ydotWheel) -> Reshape2/1  "Vy"
  SteerAng/1 -> Wheel Angles/1(SteerAng)
  r/1 -> Unary Minus/1
  VehVel/1 -> Wheel to Body Transform/1(VelVeh)
  Wheel to Body Transform/3(zdotWheel) -> Reshape5/1  "Vz"
  Unary Minus/1 -> YawRate/1
  Wheel Angles/1("WhlAng ") -> WhlAng/1, Wheel to Body Transform/2(WheelAngles)
  Reshape1/1 -> Vx/1
  Reshape2/1 -> Vy/1
  Reshape5/1 -> Vz/1
  SteerCmb/1 -> Wheel Angles/2(SteerCmb)

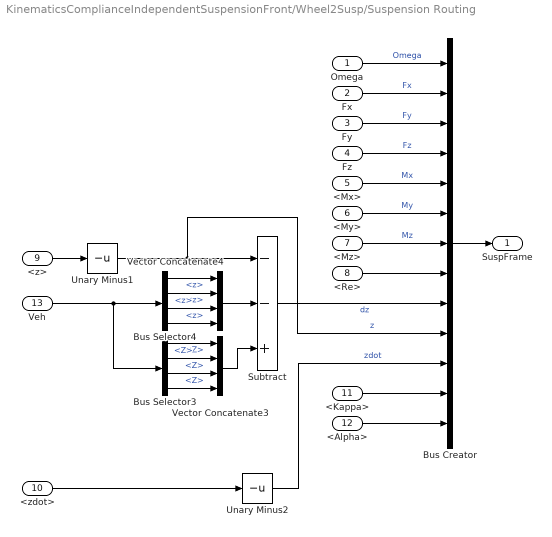
== system KinematicsComplianceIndependentSuspensionFront/Wheel2Susp/Suspension Routing ==
  Omega : Inport
  Fx : Inport  Port=2
  Fy : Inport  Port=3
  Fz : Inport  Port=4
  <Mx> : Inport  Port=5
  <My> : Inport  Port=6
  <Mz> : Inport  Port=7
  <Re> : Inport  Port=8
  <z> : Inport  Port=9
  <zdot> : Inport  Port=10
  <Kappa> : Inport  Port=11
  <Alpha> : Inport  Port=12
  Veh : Inport  Port=13
  Bus Creator : BusCreator  Inputs=13
  Bus Selector3 : BusSelector  OutputSignals=InertFrm.FrntAxl.Lft.Disp.Z,InertFrm.FrntAxl.Rght.Disp.Z,InertFrm.RearAxl.Lft.Disp.Z,InertFrm.RearAxl.Rght.Disp.Z
  Bus Selector4 : BusSelector  OutputSignals=BdyFrm.FrntAxl.Lft.Disp.z,BdyFrm.FrntAxl.Rght.Disp.z,BdyFrm.RearAxl.Lft.Disp.z,BdyFrm.RearAxl.Rght.Disp.z
  Subtract : Sum  Inputs=--+
  Unary Minus1 : UnaryMinus
  Unary Minus2 : UnaryMinus
  Vector Concatenate3 : Concatenate  NumInputs=4
  Vector Concatenate4 : Concatenate  NumInputs=4
  SuspFrame : Outport  VectorParamsAs1DForOutWhenUnconnected=off
  wires:
  <Re>/1 -> Bus Creator/8
  Unary Minus1/1 -> Subtract/1, Bus Creator/10  "z"
  Fz/1 -> Bus Creator/4  "Fz"
  <zdot>/1 -> Unary Minus2/1
  <Mz>/1 -> Bus Creator/7  "Mz"
  Unary Minus2/1 -> Bus Creator/11  "zdot"
  <z>/1 -> Unary Minus1/1
  Bus Creator/1 -> SuspFrame/1
  Fy/1 -> Bus Creator/3  "Fy"
  Omega/1 -> Bus Creator/1  "Omega"
  Fx/1 -> Bus Creator/2  "Fx"
  <Kappa>/1 -> Bus Creator/12
  <Mx>/1 -> Bus Creator/5  "Mx"
  <My>/1 -> Bus Creator/6  "My"
  <Alpha>/1 -> Bus Creator/13
  Veh/1 -> Bus Selector3/1, Bus Selector4/1
  Bus Selector3/4 -> Vector Concatenate3/4  "<Z>"
  Subtract/1 -> Bus Creator/9  "dz"
  Bus Selector4/1 -> Vector Concatenate4/1  "<z>"
  Bus Selector3/1 -> Vector Concatenate3/1  "<Z>"
  Vector Concatenate3/1 -> Subtract/3
  Vector Concatenate4/1 -> Subtract/2
  Bus Selector4/2 -> Vector Concatenate4/2  "<z>"
  Bus Selector3/3 -> Vector Concatenate3/3  "<Z>"
  Bus Selector3/2 -> Vector Concatenate3/2  "<Z>"
  Bus Selector4/4 -> Vector Concatenate4/4  "<z>"
  Bus Selector4/3 -> Vector Concatenate4/3  "<z>"

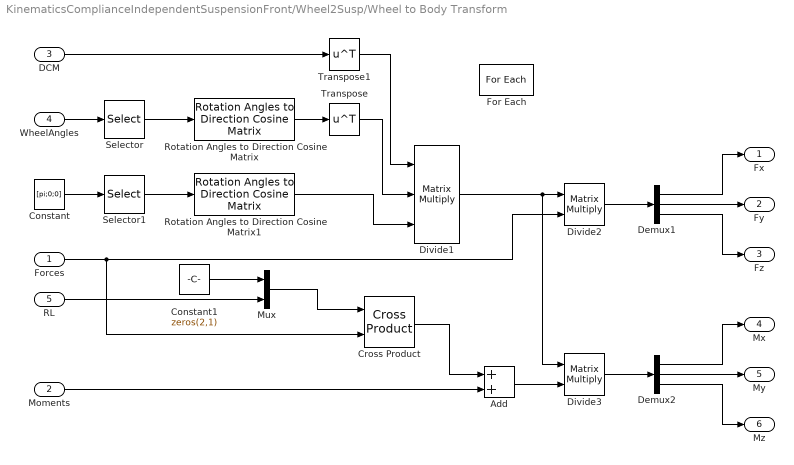
== system KinematicsComplianceIndependentSuspensionFront/Wheel2Susp/Wheel to Body Transform ==
  Forces : Inport  PortDimensions=[3,1]  Partition=on  PartitionDimension=2  PartitionWidth=1  PartitionOffset=0
  Moments : Inport  Port=2  PortDimensions=[3,1]  Partition=on  PartitionDimension=2  PartitionWidth=1  PartitionOffset=0
  DCM : Inport  Port=3  Partition=on  PartitionDimension=3  PartitionWidth=1  PartitionOffset=0
  WheelAngles : Inport  Port=4  Partition=on  PartitionDimension=2  PartitionWidth=1  PartitionOffset=0
  RL : Inport  Port=5  Partition=on  PartitionDimension=1  PartitionWidth=1  PartitionOffset=0
  Add : Sum
  Constant : Constant  Value=[pi;0;0]
  Constant1 : Constant  Value=zeros(2,1)
  Cross Product : matrix_library/Cross Product
  Demux1 : Demux  Outputs=3
  Demux2 : Demux  Outputs=3
  Divide1 : Product  Inputs=***  Multiplication=Matrix(*)
  Divide2 : Product  Inputs=**  Multiplication=Matrix(*)
  Divide3 : Product  Inputs=**  Multiplication=Matrix(*)
  For Each : ForEach  DisableCoverage=on
  Mux : Mux  Inputs=2
  Rotation Angles to Direction Cosine Matrix : autolibsharedcommon/Rotation Angles to Direction Cosine Matrix  rotationOrder=ZYX  aMode=aMode
      settings: AttributesFormatString=Rotation Order: %<rotationOrder>
  Rotation Angles to Direction Cosine Matrix1 : autolibsharedcommon/Rotation Angles to Direction Cosine Matrix  rotationOrder=ZYX  aMode=aMode
      settings: AttributesFormatString=Rotation Order: %<rotationOrder>
  Selector : Selector  InputPortWidth=3  IndexOptions=Index vector (dialog)  Indices=[3 2 1]  OutputSizes=1
  Selector1 : Selector  InputPortWidth=3  IndexOptions=Index vector (dialog)  Indices=[3 2 1]  OutputSizes=1
  Transpose : Math  Operator=transpose
  Transpose1 : Math  Operator=transpose
  Fx : Outport  ConcatenationDimension=1  VectorParamsAs1DForOutWhenUnconnected=off
  Fy : Outport  Port=2  ConcatenationDimension=1  VectorParamsAs1DForOutWhenUnconnected=off
  Fz : Outport  Port=3  ConcatenationDimension=1  VectorParamsAs1DForOutWhenUnconnected=off
  Mx : Outport  Port=4  ConcatenationDimension=1  VectorParamsAs1DForOutWhenUnconnected=off
  My : Outport  Port=5  ConcatenationDimension=1  VectorParamsAs1DForOutWhenUnconnected=off
  Mz : Outport  Port=6  ConcatenationDimension=1  VectorParamsAs1DForOutWhenUnconnected=off
  wires:
  Constant1/1 -> Mux/1
  RL/1 -> Mux/2
  Mux/1 -> Cross Product/1
  Cross Product/1 -> Add/1
  Add/1 -> Divide3/2
  Demux2/1 -> Mx/1
  Demux2/2 -> My/1
  Demux2/3 -> Mz/1
  Moments/1 -> Add/2
  Divide1/1 -> Divide2/1, Divide3/1
  Divide3/1 -> Demux2/1
  Divide2/1 -> Demux1/1
  Transpose1/1 -> Divide1/1
  DCM/1 -> Transpose1/1
  Transpose/1 -> Divide1/2
  Constant/1 -> Selector1/1
  Selector1/1 -> Rotation Angles to Direction Cosine Matrix1/1
  Rotation Angles to Direction Cosine Matrix1/1 -> Divide1/3
  Selector/1 -> Rotation Angles to Direction Cosine Matrix/1
  WheelAngles/1 -> Selector/1
  Forces/1 -> Cross Product/2, Divide2/2
  Rotation Angles to Direction Cosine Matrix/1 -> Transpose/1
  Demux1/3 -> Fz/1
  Demux1/2 -> Fy/1
  Demux1/1 -> Fx/1

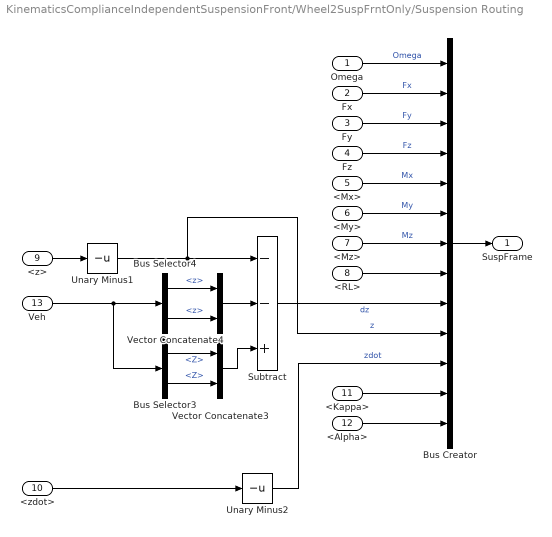
== system KinematicsComplianceIndependentSuspensionFront/Wheel2SuspFrntOnly/Suspension Routing ==
  Omega : Inport
  Fx : Inport  Port=2
  Fy : Inport  Port=3
  Fz : Inport  Port=4
  <Mx> : Inport  Port=5
  <My> : Inport  Port=6
  <Mz> : Inport  Port=7
  <RL> : Inport  Port=8
  <z> : Inport  Port=9
  <zdot> : Inport  Port=10
  <Kappa> : Inport  Port=11
  <Alpha> : Inport  Port=12
  Veh : Inport  Port=13
  Bus Creator : BusCreator  Inputs=13
  Bus Selector3 : BusSelector  OutputSignals=InertFrm.FrntAxl.Lft.Disp.Z,InertFrm.FrntAxl.Rght.Disp.Z
  Bus Selector4 : BusSelector  OutputSignals=BdyFrm.FrntAxl.Lft.Disp.z,BdyFrm.FrntAxl.Rght.Disp.z
  Subtract : Sum  Inputs=--+
  Unary Minus1 : UnaryMinus
  Unary Minus2 : UnaryMinus
  Vector Concatenate3 : Concatenate
  Vector Concatenate4 : Concatenate
  SuspFrame : Outport  VectorParamsAs1DForOutWhenUnconnected=off
  wires:
  <RL>/1 -> Bus Creator/8
  Unary Minus1/1 -> Subtract/1, Bus Creator/10  "z"
  Fz/1 -> Bus Creator/4  "Fz"
  <zdot>/1 -> Unary Minus2/1
  <Mz>/1 -> Bus Creator/7  "Mz"
  Unary Minus2/1 -> Bus Creator/11  "zdot"
  <z>/1 -> Unary Minus1/1
  Bus Creator/1 -> SuspFrame/1
  Fy/1 -> Bus Creator/3  "Fy"
  Omega/1 -> Bus Creator/1  "Omega"
  Fx/1 -> Bus Creator/2  "Fx"
  <Kappa>/1 -> Bus Creator/12
  <Mx>/1 -> Bus Creator/5  "Mx"
  <My>/1 -> Bus Creator/6  "My"
  <Alpha>/1 -> Bus Creator/13
  Veh/1 -> Bus Selector3/1, Bus Selector4/1
  Subtract/1 -> Bus Creator/9  "dz"
  Bus Selector4/1 -> Vector Concatenate4/1  "<z>"
  Bus Selector3/1 -> Vector Concatenate3/1  "<Z>"
  Vector Concatenate3/1 -> Subtract/3
  Vector Concatenate4/1 -> Subtract/2
  Bus Selector4/2 -> Vector Concatenate4/2  "<z>"
  Bus Selector3/2 -> Vector Concatenate3/2  "<Z>"

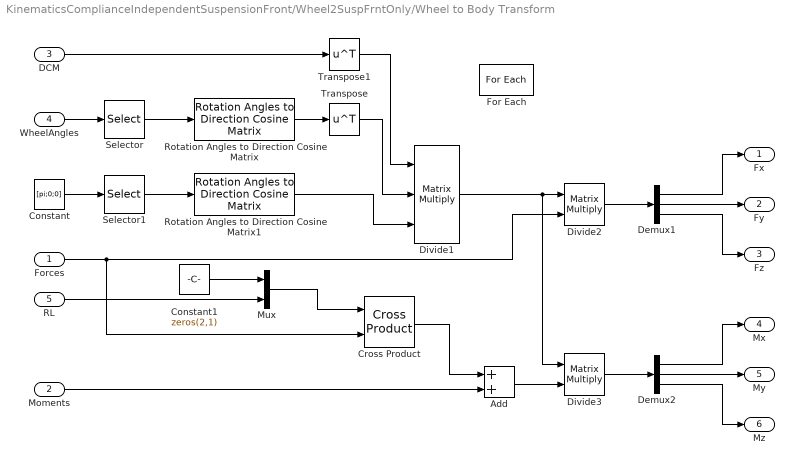
== system KinematicsComplianceIndependentSuspensionFront/Wheel2SuspFrntOnly/Wheel to Body Transform ==
  Forces : Inport  PortDimensions=[3,1]  Partition=on  PartitionDimension=2  PartitionWidth=1  PartitionOffset=0
  Moments : Inport  Port=2  PortDimensions=[3,1]  Partition=on  PartitionDimension=2  PartitionWidth=1  PartitionOffset=0
  DCM : Inport  Port=3  Partition=on  PartitionDimension=3  PartitionWidth=1  PartitionOffset=0
  WheelAngles : Inport  Port=4  Partition=on  PartitionDimension=2  PartitionWidth=1  PartitionOffset=0
  RL : Inport  Port=5  Partition=on  PartitionDimension=1  PartitionWidth=1  PartitionOffset=0
  Add : Sum
  Constant : Constant  Value=[pi;0;0]
  Constant1 : Constant  Value=zeros(2,1)
  Cross Product : matrix_library/Cross Product
  Demux1 : Demux  Outputs=3
  Demux2 : Demux  Outputs=3
  Divide1 : Product  Inputs=***  Multiplication=Matrix(*)
  Divide2 : Product  Inputs=**  Multiplication=Matrix(*)
  Divide3 : Product  Inputs=**  Multiplication=Matrix(*)
  For Each : ForEach  DisableCoverage=on
  Mux : Mux  Inputs=2
  Rotation Angles to Direction Cosine Matrix : autolibsharedcommon/Rotation Angles to Direction Cosine Matrix  rotationOrder=ZYX  aMode=aMode
      settings: AttributesFormatString=Rotation Order: %<rotationOrder>
  Rotation Angles to Direction Cosine Matrix1 : autolibsharedcommon/Rotation Angles to Direction Cosine Matrix  rotationOrder=ZYX  aMode=aMode
      settings: AttributesFormatString=Rotation Order: %<rotationOrder>
  Selector : Selector  InputPortWidth=3  IndexOptions=Index vector (dialog)  Indices=[3 2 1]  OutputSizes=1
  Selector1 : Selector  InputPortWidth=3  IndexOptions=Index vector (dialog)  Indices=[3 2 1]  OutputSizes=1
  Transpose : Math  Operator=transpose
  Transpose1 : Math  Operator=transpose
  Fx : Outport  ConcatenationDimension=1  VectorParamsAs1DForOutWhenUnconnected=off
  Fy : Outport  Port=2  ConcatenationDimension=1  VectorParamsAs1DForOutWhenUnconnected=off
  Fz : Outport  Port=3  ConcatenationDimension=1  VectorParamsAs1DForOutWhenUnconnected=off
  Mx : Outport  Port=4  ConcatenationDimension=1  VectorParamsAs1DForOutWhenUnconnected=off
  My : Outport  Port=5  ConcatenationDimension=1  VectorParamsAs1DForOutWhenUnconnected=off
  Mz : Outport  Port=6  ConcatenationDimension=1  VectorParamsAs1DForOutWhenUnconnected=off
  wires:
  Constant1/1 -> Mux/1
  RL/1 -> Mux/2
  Mux/1 -> Cross Product/1
  Cross Product/1 -> Add/1
  Add/1 -> Divide3/2
  Demux2/1 -> Mx/1
  Demux2/2 -> My/1
  Demux2/3 -> Mz/1
  Moments/1 -> Add/2
  Divide1/1 -> Divide2/1, Divide3/1
  Divide3/1 -> Demux2/1
  Divide2/1 -> Demux1/1
  Transpose1/1 -> Divide1/1
  DCM/1 -> Transpose1/1
  Transpose/1 -> Divide1/2
  Constant/1 -> Selector1/1
  Selector1/1 -> Rotation Angles to Direction Cosine Matrix1/1
  Rotation Angles to Direction Cosine Matrix1/1 -> Divide1/3
  Selector/1 -> Rotation Angles to Direction Cosine Matrix/1
  WheelAngles/1 -> Selector/1
  Forces/1 -> Cross Product/2, Divide2/2
  Rotation Angles to Direction Cosine Matrix/1 -> Transpose/1
  Demux1/3 -> Fz/1
  Demux1/2 -> Fy/1
  Demux1/1 -> Fx/1

== system KinematicsComplianceIndependentSuspensionFront/Kinematics and Compliance Independent Suspension/Calculate dynamic track width from lateral wheel center displacement change/Front Track Calculation ==
  dWhlY : Inport
  sign : Inport  Port=2
  Abs : Abs  ZeroCross=off  SaturateOnIntegerOverflow=off
  Abs1 : Abs  ZeroCross=off  SaturateOnIntegerOverflow=off
  Add : Sum  Inputs=+++
  Front Left select : Selector  InputPortWidth=4  IndexOptions=Index vector (dialog)  Indices=1  OutputSizes=1
  Front Left select1 : Selector  InputPortWidth=4  IndexOptions=Index vector (dialog)  Indices=1  OutputSizes=1
  Front Right select : Selector  InputPortWidth=4  IndexOptions=Index vector (dialog)  Indices=2  OutputSizes=1
  Front Right select1 : Selector  InputPortWidth=4  IndexOptions=Index vector (dialog)  Indices=2  OutputSizes=1
  Front Track : Constant  Value=w(1)  SampleTime=-1
  Product : Product
  Product1 : Product
  w_front : Outport
  wires:
  Front Track/1 -> Add/1
  Front Left select/1 -> Abs/1
  Front Right select/1 -> Abs1/1
  sign/1 -> Front Right select1/1, Front Left select1/1
  Product/1 -> Add/2
  Front Left select1/1 -> Product/2
  Abs1/1 -> Product1/1
  Abs/1 -> Product/1
  Product1/1 -> Add/3
  Front Right select1/1 -> Product1/2
  Add/1 -> w_front/1
  dWhlY/1 -> Front Right select/1, Front Left select/1
